simulink subsystem "Senalizacion"  (R2022b)
settings: Solver=VariableStepAuto  StartTime=0.0  StopTime=10.0  RelTol=1e-3
libraries: simulink x14, arduinolib x9
settings Model: Creator=Usuario  LastModifiedBy=Usuario

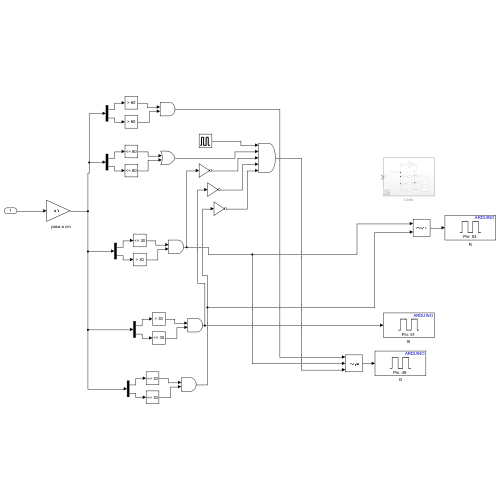
[thumbnail: Simulink's stored preview of the top-level diagram]
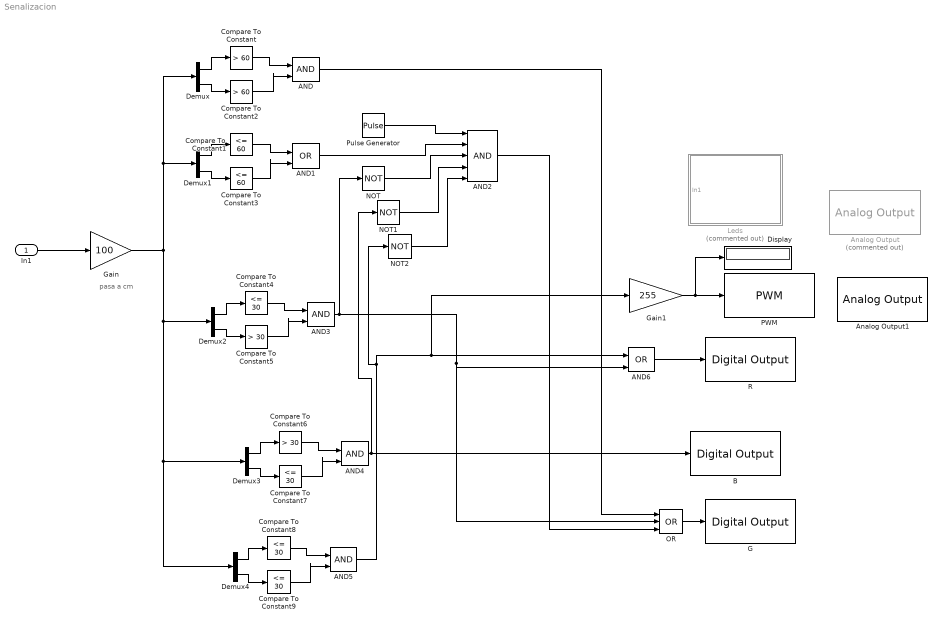
== system Senalizacion ==
  note: pasa a cm
  In1 : Inport
  AND{,3..5} (4 alike) : Logic  IconShape=distinctive  AllPortsSameDT=off  OutDataTypeStr=boolean
  AND1 : Logic  Operator=OR  IconShape=distinctive  AllPortsSameDT=off  OutDataTypeStr=boolean
  AND2 : Logic  Inputs=5  IconShape=distinctive  AllPortsSameDT=off  OutDataTypeStr=boolean
  AND6 : Logic  Operator=OR  IconShape=distinctive  AllPortsSameDT=off  OutDataTypeStr=boolean
  Analog Output : arduinolib/Analog Output  Commented=on  DACpin=DAC0  blockPlatform=arduino
  Analog Output1 : arduinolib/Analog Output  DACpin=DAC0  blockPlatform=arduino
  B : arduinolib/Digital Output  pinNumber=51  Direction=output  blockPlatform=arduino
  Compare To Constant : simulink/Logic and Bit Operations/Compare To Constant  relop=>  const=60  OutDataTypeStr=boolean
  Compare To Constant1 : simulink/Logic and Bit Operations/Compare To Constant  relop=<=  const=60  OutDataTypeStr=boolean
  Compare To Constant2 : simulink/Logic and Bit Operations/Compare To Constant  relop=>  const=60  OutDataTypeStr=boolean
  Compare To Constant3 : simulink/Logic and Bit Operations/Compare To Constant  relop=<=  const=60  OutDataTypeStr=boolean
  Compare To Constant{4,7..9} (4 alike) : simulink/Logic and Bit Operations/Compare To Constant  relop=<=  const=30  OutDataTypeStr=boolean
  Compare To Constant5 : simulink/Logic and Bit Operations/Compare To Constant  relop=>  const=30  OutDataTypeStr=boolean
  Compare To Constant6 : simulink/Logic and Bit Operations/Compare To Constant  relop=>  const=30  OutDataTypeStr=boolean
  Demux{,1..4} (5 alike) : Demux  Outputs=2
  Display : Display
  G : arduinolib/Digital Output  pinNumber=49  Direction=output  blockPlatform=arduino
  Gain : Gain  Gain=100
  Gain1 : Gain  Gain=255
  Leds : Subsystem  Commented=on
  NOT : Logic  Operator=NOT  IconShape=distinctive  AllPortsSameDT=off  OutDataTypeStr=boolean
  NOT1 : Logic  Operator=NOT  IconShape=distinctive  AllPortsSameDT=off  OutDataTypeStr=boolean
  NOT2 : Logic  Operator=NOT  IconShape=distinctive  AllPortsSameDT=off  OutDataTypeStr=boolean
  OR : Logic  Operator=OR  Inputs=3  IconShape=distinctive  AllPortsSameDT=off  OutDataTypeStr=boolean
  PWM : arduinolib/PWM  pinNumber=6  frequencyType=Default  desiredFrequency=490.2  achievableFrequency=490.2
  Pulse Generator : DiscretePulseGenerator  PulseType=Time based  Period=10  PulseWidth=0.1
  R : arduinolib/Digital Output  pinNumber=53  Direction=output  blockPlatform=arduino
  wires:
  Demux/1 -> Compare To Constant/1
  Demux/2 -> Compare To Constant2/1
  Compare To Constant/1 -> AND/1
  Compare To Constant2/1 -> AND/2
  AND/1 -> OR/1
  Demux1/1 -> Compare To Constant1/1
  Compare To Constant3/1 -> AND1/2
  Demux1/2 -> Compare To Constant3/1
  Compare To Constant1/1 -> AND1/1
  AND2/1 -> OR/3
  Demux2/1 -> Compare To Constant4/1
  Compare To Constant5/1 -> AND3/2
  Demux2/2 -> Compare To Constant5/1
  Compare To Constant4/1 -> AND3/1
  Pulse Generator/1 -> AND2/1
  AND1/1 -> AND2/2
  AND3/1 -> NOT/1, AND6/2, OR/2
  Compare To Constant6/1 -> AND4/1
  Demux3/2 -> Compare To Constant7/1
  Demux3/1 -> Compare To Constant6/1
  Compare To Constant7/1 -> AND4/2
  AND4/1 -> NOT1/1, B/1
  Demux4/2 -> Compare To Constant9/1
  Compare To Constant8/1 -> AND5/1
  Demux4/1 -> Compare To Constant8/1
  Compare To Constant9/1 -> AND5/2
  In1/1 -> Gain/1
  NOT/1 -> AND2/3
  NOT1/1 -> AND2/4
  NOT2/1 -> AND2/5
  Gain/1 -> Demux4/1, Demux3/1, Demux2/1, Demux/1, Demux1/1
  OR/1 -> G/1
  AND5/1 -> NOT2/1, AND6/1, Gain1/1
  AND6/1 -> R/1
  Gain1/1 -> PWM/1, Display/1

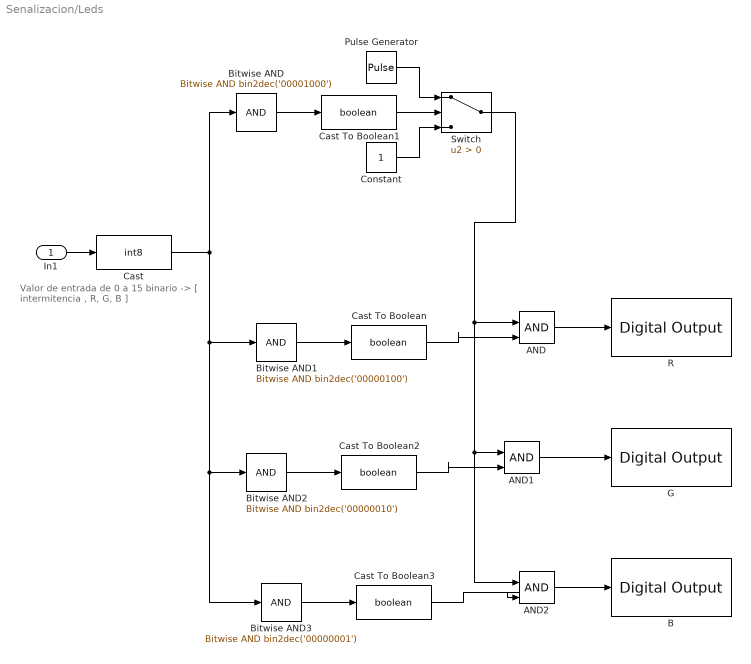
== system Senalizacion/Leds ==
  note: Valor de entrada  de 0 a 15 binario ->
      | [ intermitencia , R, G, B ]
  In1 : Inport
  AND : Logic  IconShape=distinctive  AllPortsSameDT=off  OutDataTypeStr=boolean
  AND1 : Logic  IconShape=distinctive  AllPortsSameDT=off  OutDataTypeStr=boolean
  AND2 : Logic  IconShape=distinctive  AllPortsSameDT=off  OutDataTypeStr=boolean
  B : arduinolib/Digital Output  pinNumber=51  Direction=output  blockPlatform=arduino
  Bitwise AND : simulink/Logic and Bit Operations/Bitwise Operator  logicop=AND  UseBitMask=on  BitMask=bin2dec('00001000')  BitMaskRealWorld=Stored Integer
      settings: LibrarySourceBlock=|
      | simulink/Quick Insert/Logic and Bit
      | Operations/Bitwise AND
  Bitwise AND1 : simulink/Logic and Bit Operations/Bitwise Operator  logicop=AND  UseBitMask=on  BitMask=bin2dec('00000100')  BitMaskRealWorld=Stored Integer
      settings: LibrarySourceBlock=|
      | simulink/Quick Insert/Logic and Bit
      | Operations/Bitwise AND
  Bitwise AND2 : simulink/Logic and Bit Operations/Bitwise Operator  logicop=AND  UseBitMask=on  BitMask=bin2dec('00000010')  BitMaskRealWorld=Stored Integer
      settings: LibrarySourceBlock=|
      | simulink/Quick Insert/Logic and Bit
      | Operations/Bitwise AND
  Bitwise AND3 : simulink/Logic and Bit Operations/Bitwise Operator  logicop=AND  UseBitMask=on  BitMask=bin2dec('00000001')  BitMaskRealWorld=Stored Integer
      settings: LibrarySourceBlock=|
      | simulink/Quick Insert/Logic and Bit
      | Operations/Bitwise AND
  Cast : DataTypeConversion  OutDataTypeStr=int8  SaturateOnIntegerOverflow=off  RndMeth=Floor
  Cast To Boolean{,1..3} (4 alike) : DataTypeConversion  OutDataTypeStr=boolean  SaturateOnIntegerOverflow=off  RndMeth=Floor
  Constant : Constant
  G : arduinolib/Digital Output  pinNumber=49  Direction=output  blockPlatform=arduino
  Pulse Generator : DiscretePulseGenerator  PulseType=Time based  Period=10  PulseWidth=5
  R : arduinolib/Digital Output  pinNumber=53  Direction=output  blockPlatform=arduino
  Switch : Switch  Criteria=u2 > Threshold  SaturateOnIntegerOverflow=off  InputSameDT=off
  wires:
  Cast/1 -> Bitwise AND3/1, Bitwise AND2/1, Bitwise AND1/1, Bitwise AND/1
  Pulse Generator/1 -> Switch/1
  Switch/1 -> AND2/1, AND1/1, AND/1
  Cast To Boolean2/1 -> AND1/2
  Cast To Boolean/1 -> AND/2
  Bitwise AND/1 -> Cast To Boolean1/1
  AND1/1 -> G/1
  Bitwise AND1/1 -> Cast To Boolean/1
  Cast To Boolean3/1 -> AND2/2
  Constant/1 -> Switch/3
  Bitwise AND2/1 -> Cast To Boolean2/1
  Cast To Boolean1/1 -> Switch/2
  In1/1 -> Cast/1
  AND/1 -> R/1
  AND2/1 -> B/1
  Bitwise AND3/1 -> Cast To Boolean3/1
